simulink model "untitled"  (R2018b)
settings: Solver=VariableStepAuto  StartTime=0.0  StopTime=30.0  RelTol=1e-3
settings Model: Creator=zhele  LastModifiedBy=zhele

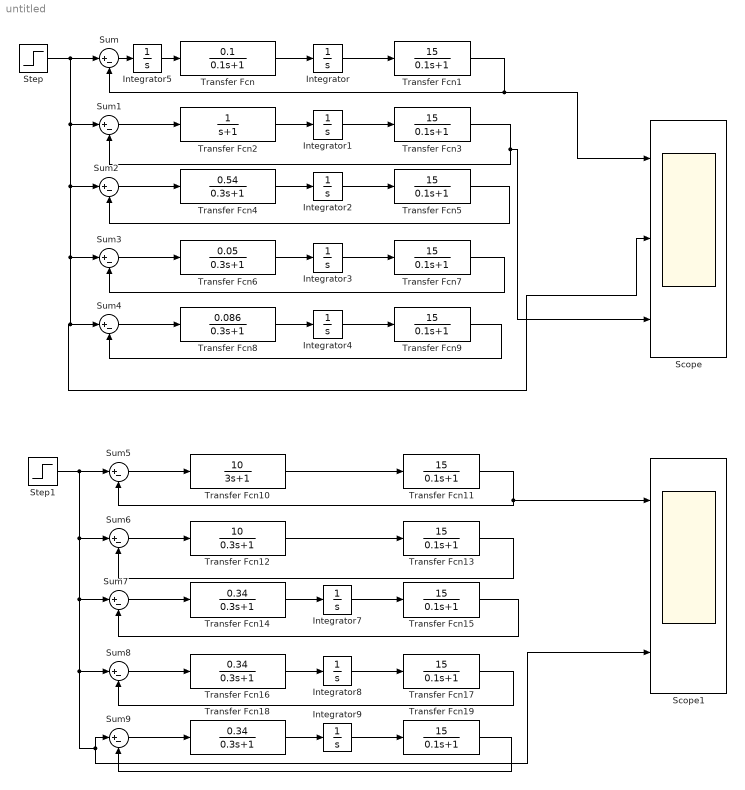
== system untitled ==
  Integrator{,1..5,7..9} (9 alike) : Integrator
  Scope : Scope  NumInputPorts=3
  Scope1 : Scope  NumInputPorts=3
  Step : Step  SampleTime=0
  Step1 : Step  SampleTime=0
  Sum{,1..9} (10 alike) : Sum  Inputs=|+-
  Transfer Fcn : TransferFcn  Numerator=[0.1]  Denominator=[0.1 1]
  Transfer Fcn{1,3,5,7,9,11,13,15,17,19} (10 alike) : TransferFcn  Numerator=[15]  Denominator=[0.1 1]
  Transfer Fcn10 : TransferFcn  Numerator=[10]  Denominator=[3 1]
  Transfer Fcn12 : TransferFcn  Numerator=[10]  Denominator=[0.3 1]
  Transfer Fcn14 : TransferFcn  Numerator=[0.34]  Denominator=[0.3 1]
  Transfer Fcn16 : TransferFcn  Numerator=[0.34]  Denominator=[0.3 1]
  Transfer Fcn18 : TransferFcn  Numerator=[0.34]  Denominator=[0.3 1]
  Transfer Fcn2 : TransferFcn  Denominator=[1 1]
  Transfer Fcn4 : TransferFcn  Numerator=[0.54]  Denominator=[0.3 1]
  Transfer Fcn6 : TransferFcn  Numerator=[0.05]  Denominator=[0.3 1]
  Transfer Fcn8 : TransferFcn  Numerator=[0.086]  Denominator=[0.3 1]
  wires:
  Transfer Fcn/1 -> Integrator/1
  Integrator/1 -> Transfer Fcn1/1
  Transfer Fcn1/1 -> Sum/2, Scope/1
  Integrator1/1 -> Transfer Fcn3/1
  Transfer Fcn2/1 -> Integrator1/1
  Sum1/1 -> Transfer Fcn2/1
  Transfer Fcn3/1 -> Scope/3, Sum1/2
  Integrator2/1 -> Transfer Fcn5/1
  Transfer Fcn4/1 -> Integrator2/1
  Sum2/1 -> Transfer Fcn4/1
  Integrator3/1 -> Transfer Fcn7/1
  Transfer Fcn6/1 -> Integrator3/1
  Sum3/1 -> Transfer Fcn6/1
  Transfer Fcn5/1 -> Sum2/2
  Transfer Fcn7/1 -> Sum3/2
  Integrator4/1 -> Transfer Fcn9/1
  Sum4/1 -> Transfer Fcn8/1
  Transfer Fcn8/1 -> Integrator4/1
  Transfer Fcn9/1 -> Sum4/2
  Transfer Fcn15/1 -> Sum7/2
  Sum7/1 -> Transfer Fcn14/1
  Transfer Fcn14/1 -> Integrator7/1
  Transfer Fcn13/1 -> Sum6/2
  Integrator7/1 -> Transfer Fcn15/1
  Transfer Fcn12/1 -> Transfer Fcn13/1
  Sum6/1 -> Transfer Fcn12/1
  Transfer Fcn19/1 -> Sum9/2
  Sum9/1 -> Transfer Fcn18/1
  Integrator9/1 -> Transfer Fcn19/1
  Transfer Fcn10/1 -> Transfer Fcn11/1
  Integrator8/1 -> Transfer Fcn17/1
  Sum8/1 -> Transfer Fcn16/1
  Transfer Fcn16/1 -> Integrator8/1
  Transfer Fcn17/1 -> Sum8/2
  Sum5/1 -> Transfer Fcn10/1
  Transfer Fcn11/1 -> Sum5/2, Scope1/1
  Transfer Fcn18/1 -> Integrator9/1
  Step/1 -> Scope/2, Sum4/1, Sum3/1, Sum2/1, Sum1/1, Sum/1
  Step1/1 -> Scope1/3, Sum9/1, Sum8/1, Sum7/1, Sum6/1, Sum5/1
  Sum/1 -> Integrator5/1
  Integrator5/1 -> Transfer Fcn/1
